simulink model "ControlObject"  (R2023a)
settings: Solver=VariableStepAuto  StartTime=0.0  StopTime=10.0  RelTol=1e-3
settings Model: Creator=romav  LastModifiedBy=romav

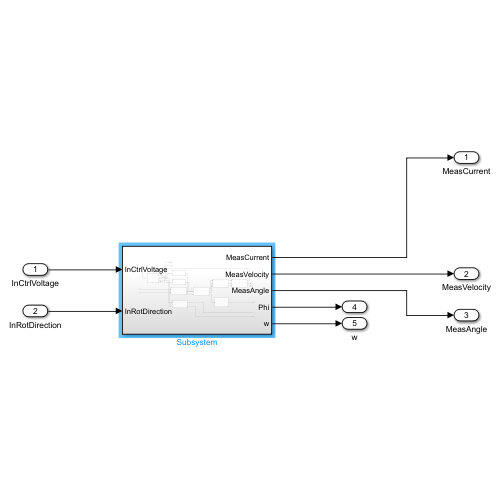
[thumbnail: Simulink's stored preview of the top-level diagram]
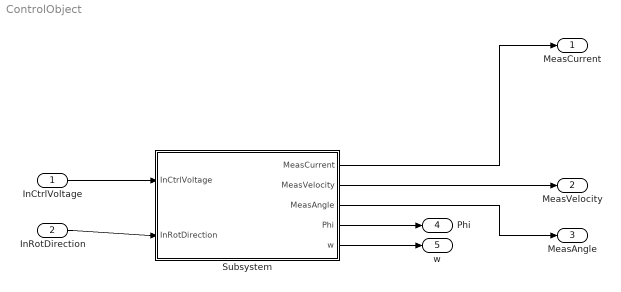
== system ControlObject ==
  InCtrlVoltage : Inport
  InRotDirection : Inport  Port=2
  Subsystem : Subsystem
  MeasCurrent : Outport
  MeasVelocity : Outport  Port=2
  MeasAngle : Outport  Port=3
  " Phi" : Outport  Port=4
  w : Outport  Port=5
  wires:
  InCtrlVoltage/1 -> Subsystem/1(InCtrlVoltage)
  InRotDirection/1 -> Subsystem/2(InRotDirection)
  Subsystem/1(MeasCurrent) -> MeasCurrent/1
  Subsystem/2(MeasVelocity) -> MeasVelocity/1
  Subsystem/3(MeasAngle) -> MeasAngle/1
  Subsystem/4(" Phi") -> " Phi"/1
  Subsystem/5(w) -> w/1

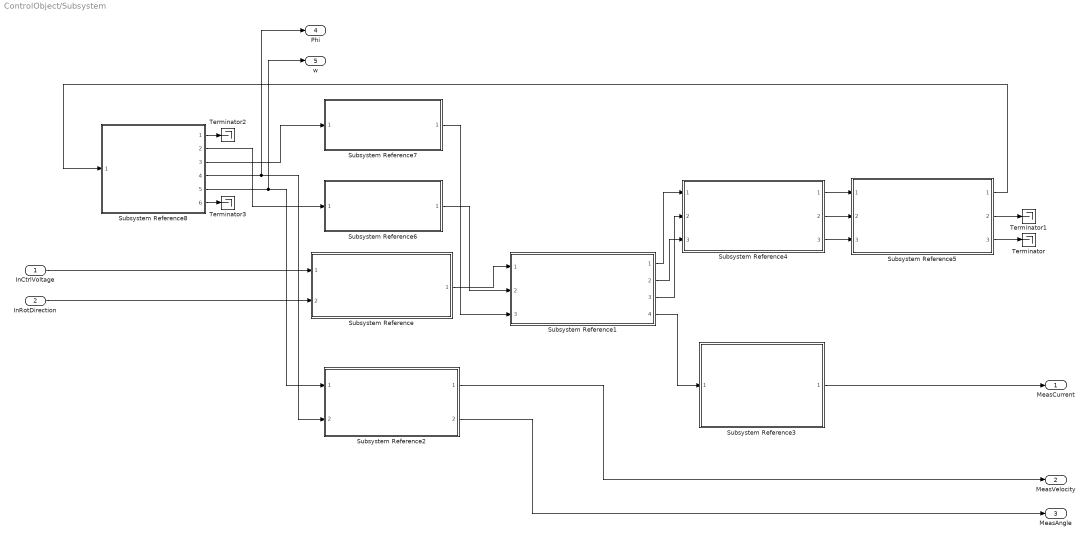
== system ControlObject/Subsystem ==
  InCtrlVoltage : Inport
  InRotDirection : Inport  Port=2
  Subsystem Reference : Subsystem  ReferencedSubsystem=Power_Gain  Kpa=7.3
  Subsystem Reference1 : Subsystem  ReferencedSubsystem=Motor  kw=62.8  km=16e-3  motor_nominal_voltage=24  vis_friction_coef_motor=0.1
  Subsystem Reference2 : Subsystem  ReferencedSubsystem=HallSensor
  Subsystem Reference3 : Subsystem  ReferencedSubsystem=CurrentSensor
  Subsystem Reference4 : Subsystem  ReferencedSubsystem=Reductor  i_gear=100  J_gear=2.4e-6  vis_friction_coef_gear=0.15
  Subsystem Reference5 : Subsystem  ReferencedSubsystem=RackAndPinion  i_rp=20000  vis_friction_coef_rp=0.002  J_pinion=1e-6
  Subsystem Reference6 : Subsystem  ReferencedSubsystem=BackwardAccConverter
  Subsystem Reference7 : Subsystem  ReferencedSubsystem=BackwardAccConverter
  Subsystem Reference8 : Subsystem  ReferencedSubsystem=InversePendulum
  Terminator{,1..3} (4 alike) : Terminator
  MeasCurrent : Outport
  MeasVelocity : Outport  Port=2
  MeasAngle : Outport  Port=3
  " Phi" : Outport  Port=4
  w : Outport  Port=5
  wires:
  Subsystem Reference8/3 -> Subsystem Reference7/1
  Subsystem Reference8/1 -> Terminator2/1
  Subsystem Reference1/1 -> Subsystem Reference4/1
  Subsystem Reference8/4 -> " Phi"/1, Subsystem Reference2/2
  Subsystem Reference4/2 -> Subsystem Reference5/2
  Subsystem Reference1/3 -> Subsystem Reference4/2
  Subsystem Reference7/1 -> Subsystem Reference1/3
  Subsystem Reference4/3 -> Subsystem Reference5/3
  Subsystem Reference1/2 -> Subsystem Reference4/3
  Subsystem Reference1/4 -> Subsystem Reference3/1
  Subsystem Reference8/5 -> w/1, Subsystem Reference2/1
  InCtrlVoltage/1 -> Subsystem Reference/1
  Subsystem Reference2/1 -> MeasVelocity/1
  Subsystem Reference4/1 -> Subsystem Reference5/1
  Subsystem Reference/1 -> Subsystem Reference1/1
  Subsystem Reference5/2 -> Terminator1/1
  Subsystem Reference5/3 -> Terminator/1
  Subsystem Reference6/1 -> Subsystem Reference1/2
  InRotDirection/1 -> Subsystem Reference/2
  Subsystem Reference3/1 -> MeasCurrent/1
  Subsystem Reference2/2 -> MeasAngle/1
  Subsystem Reference8/2 -> Subsystem Reference6/1
  Subsystem Reference5/1 -> Subsystem Reference8/1
  Subsystem Reference8/6 -> Terminator3/1
